simulink model "fik_gimbal_two"  (R2016a)
settings: Solver=VariableStepAuto  StartTime=0.0  StopTime=10.0  RelTol=1e-3
values from neighbouring files (symbols this model uses):
  A_k = -eye(3)    [transfer_ks_init.m]
  B_k = eye(3)    [transfer_ks_init.m]
  P = eye(3)    [transfer_ks_init.m]
undefined symbols (not defined in the file or in its folder): transfer_ks_init
libraries: aerolibtransform2 x3, aerolibutil x1
settings Model: Creator=glenn  LastModifiedBy=glenn
settings GRTTargetCC: GeneratePreprocessorConditionals=Use local settings

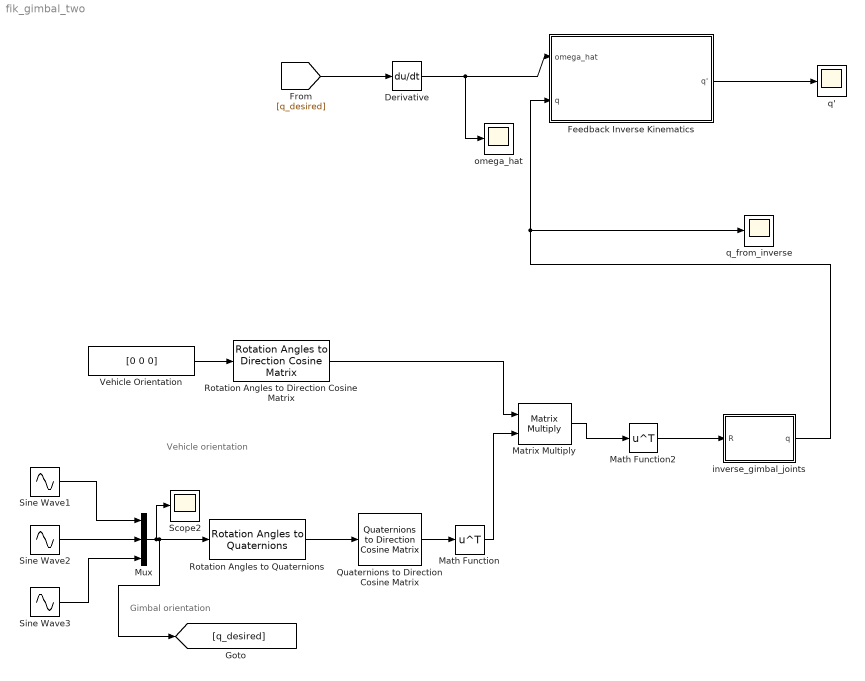
== system fik_gimbal_two ==
  note: Vehicle orientation
  note: Gimbal orientation
  Derivative : Derivative
  Feedback Inverse Kinematics : Subsystem
  Math Function : Math  Operator=transpose  SaturateOnIntegerOverflow=on
  Math Function2 : Math  Operator=transpose  SaturateOnIntegerOverflow=on
  Matrix Multiply : Product  Multiplication=Matrix(*)
  Mux : Mux  Inputs=3
  Quaternions to Direction Cosine Matrix : aerolibtransform2/Quaternions to  Direction Cosine Matrix
  Rotation Angles to Direction Cosine Matrix : aerolibtransform2/Rotation Angles to Direction Cosine Matrix  rotationOrder=ZYX
  Rotation Angles to Quaternions : aerolibtransform2/Rotation Angles to Quaternions  rotationOrder=ZXZ
  Scope2 : Scope
  Sine Wave1 : Sin  Amplitude=pi  SampleTime=0
  Sine Wave2 : Sin  Amplitude=pi/2  Bias=pi/2  SampleTime=0
  Sine Wave3 : Sin  Amplitude=pi/2  Bias=-pi/2  SampleTime=0
  Vehicle Orientation : Constant  Value=[0 0 0]
  inverse_gimbal_joints : MATLAB Function  TreatAsAtomicUnit=on
  omega_hat : Scope
  q' : Scope
  q_from_inverse : Scope
  wires:
  Derivative/1 -> omega_hat/1, Feedback Inverse Kinematics/1(omega_hat)
  Feedback Inverse Kinematics/1(q') -> q'/1
  Mux/1 -> Rotation Angles to Quaternions/1, [q_desired], Scope2/1
  Rotation Angles to Quaternions/1 -> Quaternions to Direction Cosine Matrix/1
  Vehicle Orientation/1 -> Rotation Angles to Direction Cosine Matrix/1
  Matrix Multiply/1 -> Math Function2/1
  Quaternions to Direction Cosine Matrix/1 -> Math Function/1
  Math Function/1 -> Matrix Multiply/2
  Rotation Angles to Direction Cosine Matrix/1 -> Matrix Multiply/1
  Sine Wave1/1 -> Mux/1
  Sine Wave2/1 -> Mux/2
  Sine Wave3/1 -> Mux/3
  Math Function2/1 -> inverse_gimbal_joints/1(R)
  inverse_gimbal_joints/1(q) -> Feedback Inverse Kinematics/2(q), q_from_inverse/1
  [q_desired] -> Derivative/1

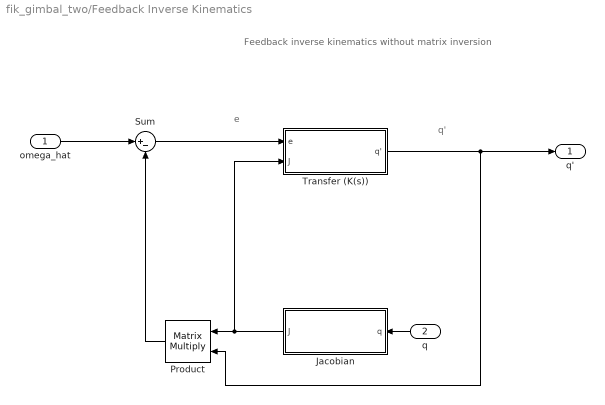
== system fik_gimbal_two/Feedback Inverse Kinematics ==
  note: e
  note: q'
  note: Feedback inverse kinematics without matrix inversion
  omega_hat : Inport
  q : Inport  Port=2
  Jacobian : Subsystem
  Product : Product  Multiplication=Matrix(*)
  Sum : Sum  Inputs=|+-
  Transfer (K(s)) : Subsystem  InitFcn=transfer_ks_init;
  q' : Outport
  wires:
  Jacobian/1(J) -> Product/1, Transfer (K(s))/2(J)
  omega_hat/1 -> Sum/1
  Transfer (K(s))/1(q') -> Product/2, q'/1
  Sum/1 -> Transfer (K(s))/1(e)
  q/1 -> Jacobian/1(q)
  Product/1 -> Sum/2

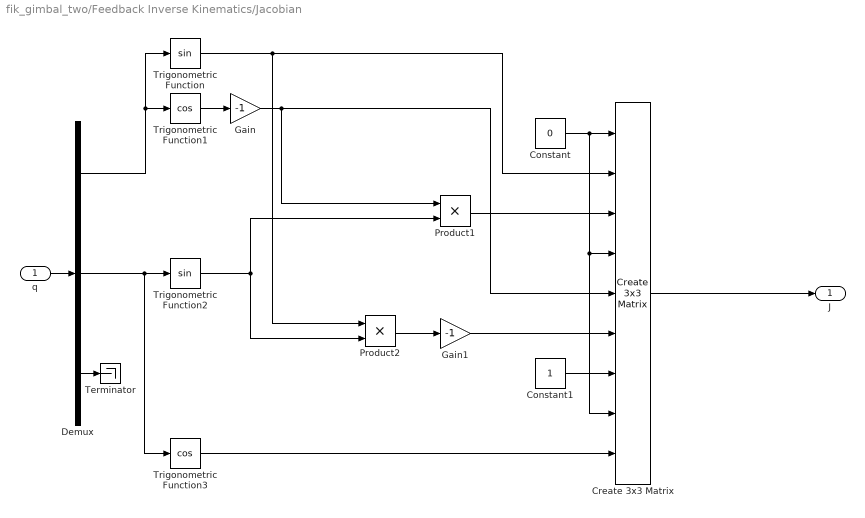
== system fik_gimbal_two/Feedback Inverse Kinematics/Jacobian ==
  q : Inport
  Constant : Constant  Value=0
  Constant1 : Constant
  Create 3x3 Matrix : aerolibutil/Create 3x3 Matrix
  Demux : Demux  Outputs=3
  Gain : Gain  Gain=-1
  Gain1 : Gain  Gain=-1
  Product1 : Product
  Product2 : Product
  Terminator : Terminator
  Trigonometric Function : Trigonometry
  Trigonometric Function1 : Trigonometry  Operator=cos
  Trigonometric Function2 : Trigonometry
  Trigonometric Function3 : Trigonometry  Operator=cos
  J : Outport
  wires:
  q/1 -> Demux/1
  Demux/1 -> Trigonometric Function/1, Trigonometric Function1/1
  Create 3x3 Matrix/1 -> J/1
  Constant/1 -> Create 3x3 Matrix/8, Create 3x3 Matrix/4, Create 3x3 Matrix/1
  Constant1/1 -> Create 3x3 Matrix/7
  Trigonometric Function/1 -> Product2/1, Create 3x3 Matrix/2
  Trigonometric Function1/1 -> Gain/1
  Gain/1 -> Product1/1, Create 3x3 Matrix/5
  Demux/2 -> Trigonometric Function3/1, Trigonometric Function2/1
  Trigonometric Function2/1 -> Product2/2, Product1/2
  Product1/1 -> Create 3x3 Matrix/3
  Product2/1 -> Gain1/1
  Gain1/1 -> Create 3x3 Matrix/6
  Trigonometric Function3/1 -> Create 3x3 Matrix/9
  Demux/3 -> Terminator/1

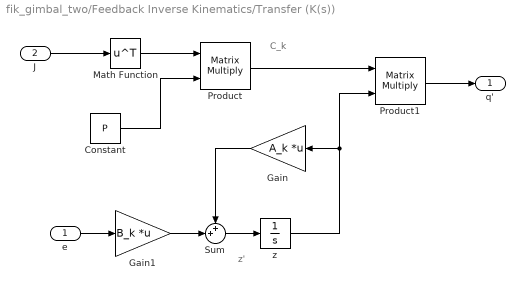
== system fik_gimbal_two/Feedback Inverse Kinematics/Transfer (K(s)) ==
  note: C_k
  note: z'
  e : Inport
  J : Inport  Port=2
  Constant : Constant  Value=P
  Gain : Gain  Gain=A_k  Multiplication=Matrix(K*u)
  Gain1 : Gain  Gain=B_k  Multiplication=Matrix(K*u)
  Math Function : Math  Operator=transpose  SaturateOnIntegerOverflow=on
  Product : Product  Multiplication=Matrix(*)
  Product1 : Product  Multiplication=Matrix(*)
  Sum : Sum  Inputs=++|
  z : Integrator
  q' : Outport
  wires:
  z/1 -> Gain/1, Product1/2
  Gain/1 -> Sum/1
  Sum/1 -> z/1
  e/1 -> Gain1/1
  Gain1/1 -> Sum/2
  J/1 -> Math Function/1
  Math Function/1 -> Product/1
  Constant/1 -> Product/2
  Product/1 -> Product1/1
  Product1/1 -> q'/1

== matlab function fik_gimbal_two/inverse_gimbal_joints ==
  data: R input; q output
function q = fcn(R)
%#codegen

    theta = 0;
    phi = 0;
    psi = 0;

    USE_POSITIVE_PITCH = true;

    if ( ~(is_zero(R(1,3))) || ~(is_zero(R(2,3))))
        if (USE_POSITIVE_PITCH)
            theta = atan2(R(3,3), sqrt(1-R(3,3)^2));
            phi = atan2(R(1,3), R(2,3));
            psi = atan2(-R(3,1),R(3,2));
        else
            theta = atan2(R(3,3), -sqrt(1-R(3,3)^2));
            phi = atan2(-R(1,3), -R(2,3));
            psi = atan2(R(3,1), -R(3,2));
        end
    else
        if (R(3,3) > 0)
            sum_phi_psi = atan2(R(1,1),R(2,1));
            phi = 0; % Some convention?
            psi = sum_phi_psi - phi;
            theta = 0;
        else
            difference_phi_psi = atan2(-R(1,1), -R(1,2));
            phi = 0; % Some convention
            psi = phi - difference_phi_psi;
            theta = pi;
        end
    end
    
    q = [phi; theta; psi];
end
    
function [ zero ] = is_zero(number)

    DELTA = 1e-5;

    if (abs(number) <= DELTA)
        zero = true;
    else
        zero = false;
    end
end
